simulink model "ForceMomentCBAgent2"  (Simulink 7.1)
settings: Solver=ode45  SolverMode=SingleTasking  StartTime=0.0  StopTime=10.0  RelTol=1e-3  AbsTol=1e-6
settings Model: Creator=The MathWorks Inc.  LastModifiedBy=suarezjl  ExtModeTrigMode=oneshot  ExtModeArmWhenConnect=off  ExtModeAutoUpdateStatusClock=off
settings DataIOCC: LimitDataPoints=off  SignalLoggingName=logsOut
settings OptimizationCC: BooleanDataType=off  InlineInvariantSignals=on
settings DebuggingCC: SaveWithParameterizedLinksMsg=none  CheckExecutionContextPreStartOutputMsg=on  CheckExecutionContextRuntimeOutputMsg=on  SignalResolutionControl=TryResolveAllWithWarning  SolverPrmCheckMsg=none  MultiTaskDSMMsg=warning  MultiTaskCondExecSysMsg=none  IntegerOverflowMsg=none  StrictBusMsg=None
settings HardwareCC: TargetUnknown=on
settings ModelReferenceCC: UpdateModelReferenceTargets=IfOutOfDate
settings RTWCC: IncludeERTFirstTime=on
settings GRTTargetCC: TargetFcnLib=ansi_tfl_tmw.mat

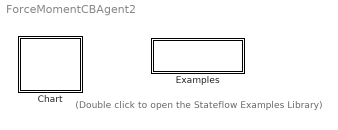
== system ForceMomentCBAgent2 ==
  note: (Double click to open the
      | Stateflow Examples Library)
  Chart : Stateflow chart
  Examples : Subsystem
      settings: OpenFcn=sf('Private','sf_examples')
      mask Display: disp('Examples')

== system ForceMomentCBAgent2/Examples ==

== stateflow chart Chart ==
  state Initialize
    \\Octavia\ISACControlBasisModule\RightModule\Arm\ArmController.DoHomingRoutine()
    \\Octavia\ISACControlBasisModule\ForceCB\StateMachine.Wait(5000)
    \\Octavia\ISACControlBasisModule\RightModule\Arm\InverseKinematics.Initialize()
    \\Octavia\ISACControlBasisModule\ForceCB\ForceCB.Initialize()
  state ControlBasis
    \\Octavia\ISACControlBasisModule\RightModule\Arm\ArmController.Move()
    \\Octavia\ISACControlBasisModule\ForceCB\ForceCB.ComputeControlBasis()
  state Stop
    \\Octavia\ISACControlBasisModule\RightModule\Arm\ArmController.DoHomingRoutine()
    \\Octavia\ISACControlBasisModule\ForceCB\StateMachine.Wait(5000)
    \\Octavia\ISACControlBasisModule\RightModule\ForceSensor\StateMachine.Stop()
  state StartStateMachines
    \\Octavia\ISACControlBasisModule\RightModule\ForceSensor\StateMachine.LoadSM()
    \\Octavia\ISACControlBasisModule\RightModule\ForceSensor\StateMachine.Start()
  state Close
    \\Octavia\ISACControlBasisModule\RightModule\Arm\ArmController.Close()
    \\Octavia\ISACControlBasisModule\ForceCB\StateMachine.Wait(5000)
    \\Octavia\ISACControlBasisModule\RightModule\ForceSensor\ATISensor.Close()
  (default) -> Initialize : Start
  Initialize -> StartStateMachines : Always
  ControlBasis -> ControlBasis [order 2] : Default
  ControlBasis -> Stop [order 3] : Signal="Stop"
  StartStateMachines -> ControlBasis : Always
  Stop -> Close : Signal="Close"
  ControlBasis -> Close [order 1] : Signal="Close"
